simulink model "narmaL2"  (R2017a)
settings: Solver=ode45  StartTime=0.0  StopTime=600  RelTol=1e-3  AbsTol=1e-8  EnableMultiTasking=on
undefined symbols (not defined in the file): Ar, hmax, k12, k2, qmax, qmin
libraries: neural x1
settings Model: Creator=Adolfo  LastModifiedBy=bad
settings DataIOCC: LimitDataPoints=on  SaveFormat=Array  SignalLoggingSaveFormat=ModelDataLogs
settings OptimizationCC: ExpressionDepthLimit=2147483647  InitFltsAndDblsToZero=on  LifeSpan=inf
settings DebuggingCC: SaveWithParameterizedLinksMsg=none  UnderspecifiedInitializationDetection=Classic  MergeDetectMultiDrivingBlocksExec=none  SignalResolutionControl=TryResolveAllWithWarning  SolverPrmCheckMsg=warning  MultiTaskDSMMsg=warning  MultiTaskCondExecSysMsg=none  FcnCallInpInsideContextMsg=warning  StateNameClashWarn=warning  SFUnexpectedBacktrackingDiag=warning  SFNoUnconditionalDefaultTransitionDiag=warning  SFExecutionAtInitializationDiag=none
settings HardwareCC: ProdBitPerPointer=32  ProdBitPerSizeT=32  ProdBitPerPtrDiffT=32  ProdLargestAtomicFloat=None  ProdIntDivRoundTo=Undefined  ProdEndianess=Unspecified  ProdWordSize=32  ProdHWDeviceType=32-bit Generic
settings ModelReferenceCC: PropagateSignalLabelsOutOfModel=off
settings GRTTargetCC: TargetFcnLib=ansi_tfl_tmw.mat  TargetLangStandard=C89/C90 (ANSI)  GeneratePreprocessorConditionals=Disable all  CombineOutputUpdateFcns=off  GRTInterface=on
settings ConfigComp: CovMetricSettings=dw  CovHtmlReporting=on  CovSaveCumulativeToWorkspaceVar=on  CovSaveSingleToWorkspaceVar=on  CovExternalEMLEnable=off

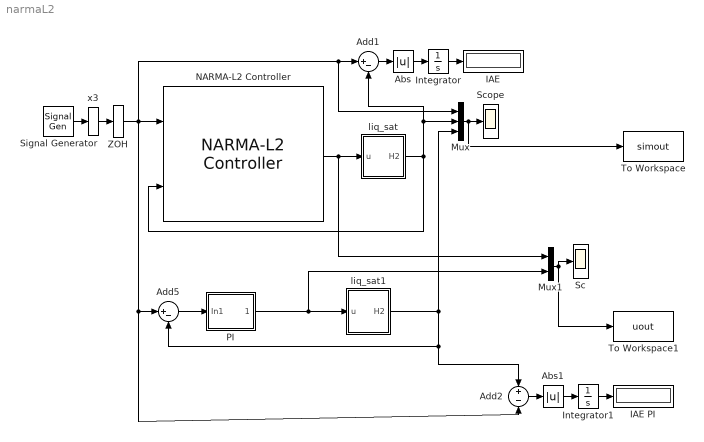
== system narmaL2 ==
  Abs : Abs
  Abs1 : Abs
  Add1 : Sum  Inputs=|+-
  Add2 : Sum  Inputs=+-
  Add5 : Sum  Inputs=|+-
  IAE : Display
  IAE PI : Display
  Integrator : Integrator
  Integrator1 : Integrator
  Mux : Mux  Inputs=3
  Mux1 : Mux  Inputs=2
  NARMA-L2 Controller : neural/Control Systems/NARMA-L2 Controller  Normalize=0  IW1_1=[0.82460127400622895699 0.8896463368737389521 0.68546670272826126791 0.40062646320525224786 -0.25514938442817886033 -1.0240928312478898565 0.01985610351462809009 -0.46086785635635324487 0.94631219312424474932;0.036728497037354770893 0.19820587025539637693 0.5134046067190429774 -0.28308665590364079367 0.16634615705465116697 -0.19327214150223945288 0.44626445203043108023 -0.37497664913527994912 -1.2593297879998377464;0.17045653362356394389 0.023322745585506728799 -0.16838760773330646581 -0.10701132675338295708 0.010654227345909813435 0.1449966612244368569 -0.17756301718275338541 -0.18227958909014374544 -0.38348992703727546871;0.12615415324788967211 -0.18534569723836363808 -1.0200895437469548188 0.76838532857597940939 0.98097883267960284126 -0.21973584499459244967 0.03310600597960997038 0.069654714512501686441 -0.14027211700811134665;0.1320897113109678056 0.31680147111401896209 0.25021595234304006006 -0.016525321314774212705 -0.21919505774665110076 -0.37402348708549482126 -1.0968105491481070501 0.91582443973852623031 0.0044695347566739282094;-0.7988884883001775572 0.77582113437411803769 -0.60287216812896193829 -0.36912054169125485537 0.21145344175312599799 0.041615517227819698309 -0.085528912678096744027 -0.087132152123573891611 0.22015982561206209889;0.38811289402447946006 -0.47324853510461034611 -0.3049238130253699719 0.18104699279980657201 -0.043398814371963738423 1.5082749992737731759 -0.21608774779125763943 -0.2687124972395262823 0.054263947622901022305;1.1246575579809743317 -1.4157437079060470886 0.50688303082942087752 -0.11200608235320431982 -0.019230053512198676258 0.039154841142778194774 -0.020848842953317365395 -0.0039643054993909083994 0.0021401530759821811578;-0.33909893220812831194 0.50899750059057413676 -0.11735584324002928946 -0.019827280110979929317 0.032300329714020560579 -0.024097353999024410248 0.010017402098296960752 0.0026810266030865173396 -0.0014331156384576751797;-1.0805049007907001624 -0.70717796914684893927 0.080234787439031840517 -0.024130003005768181634 0.61532233525059065737 -0.78459118241978287323 -0.35469066371022112127 0.26370174065851531564 0.96317052346297893362;1.9740765052747122343 -1.3610397597231203015 -1.0022880825653401882 -1.0625792463000296451 0.39565868260919517807 1.0051796856926122903 -0.093110283049667660893 0.082619795370768994713 0.016167328722534651808;-0.099469418461439612633 -0.40278027465848725841 -0.47089352901982867161 0.067031861646037194102 0.067547876656573649368 -0.25337998905188230392 0.96800361382420307965 0.45478805765030561048 -0.88698458107894961877;-1.4529527791908256606 0.1568067925322553513 -1.0986307740376015651 0.50153125106809171019 1.8691578273410005551 -0.79110151965966046816 0.73146402793697962164 0.022439777516628570814 0.020810924991256300742;-0.50900373914479313253 0.45814995583261830525 1.1456276180888709249 -1.5430241957026751276 -1.1310824923962929933 1.6740042919720710124 0.0049835931941092440067 -0.21304497923218682076 0.22522168568231107355;-0.37853429671826843705 0.37147006156279560596 -0.039743427633454841974 -0.061152055209479534714 0.042323568373044434532 -0.030245584846645769822 0.0069853908900416143701 0.003085405104233879172 -0.0018039537708811155189]  IW3_2=[-0.0097959372062227899336 0.50164014031742043542 0.63468394272614803153 0.43785446437782760132 -0.85838662096177431593 -1.6429674363166957285 0.18620560020054865991 -0.20320963371365138861 0.1422464600996860562;0.61697123621765026513 -0.88474969392431768167 -0.17864680986586969902 0.57991588808705751834 -0.49305615632303451124 -0.14794008742070452467 -0.03381079823533119505 0.19828324754626353021 -0.13441497495430421161;0.75398603138863662387 -0.48502308801037824493 0.003517610550923244532 0.26274238746623168606 1.5420625628861919232 0.63856894885611914514 -0.96123455216385822464 0.36018548400164290824 0.27701194349752655821;-0.91051269616708951915 -0.33958428131669032846 0.95290714037654755675 0.073612967304474821728 0.20996630936475935147 -0.11065462514984893139 0.077052212643874129494 0.01070943416917579695 -0.012385540173234274586;0.16443588781347087679 0.67006770786870961665 0.6884708055347915634 0.12870790339816937098 -0.41100084195716968249 0.15755452730655974958 -0.73654367631738970612 0.68488352611535630032 0.12549502724547745292;0.96063218759521951107 0.42758867397607214222 -1.2651835130708153354 -0.71554516783911048528 0.33759670629329363578 3.0872236638658465679 -0.25695606251724467661 -0.6782830882585768606 0.30962652904977577828;0.46706721394832628746 0.55353287601559852948 0.69911433634345299115 -0.847525649008489812 -0.25054686095300104931 0.14274435057194184706 -0.18615252503951984497 0.043140727653120047869 0.018608224525331850535;0.8450107012365678516 -1.0798938373582389616 0.4910317222187983166 -0.86347129900768826438 1.0710687752896397296 0.43791333647511820892 0.19374518879967442264 0.075971376265251508442 -0.26660867173805530284;-1.1018119121817588901 -1.4733616883621358795 1.6692288626171432053 0.21358701221124865022 0.043292338661919220477 0.68525051125483049663 0.17902788630519350654 0.23583551788146939199 -0.067173883509847112649;-1.6739081117719991632 1.1177760431219634363 0.47132218615963206165 0.71906947248461727806 -0.42506946994967831355 -2.6242730123560318312 -0.069469553526874824878 0.36308679776155350361 -0.093452349928687061809;-0.77782044035700470541 1.3269413258585924797 -0.43742364026979768665 -0.023010647734847556461 0.017468313680051351239 -0.0088931212673651737627 0.015187382276087291189 0.0036293475455048841011 -0.002197602546328692244;0.11474360757461192495 0.17241811619609576089 -0.19699798228017731394 -0.41145992998582819888 0.37195555743245412028 0.78015868587050629657 0.25978078167190638004 -0.052543511873452151961 -0.25085985498759311163;0.19472679919234092694 0.063155605684590970794 0.13947613217810500563 0.42627460857168703035 0.68910375257047229436 0.43623001225915630785 -0.11874103010955096293 -0.64467095432470289396 0.48229399541859729883;-0.24262201049709156142 -0.95726247674483733174 -0.31738687796607734093 0.56125633081053638573 0.18291069266519230374 0.78624661233304093955 0.16104772558408494976 -0.12893771517534594051 0.085536694064360610512;-0.55990960267259715089 -0.53748643019794273279 -0.63104960549687771909 -0.32569970560154087869 1.0555322514736951156 1.9557692781627589174 0.025912193569968444001 -0.18764326359315686155 0.24956092961725520607]  IW5_3=0.68524973220823459652  LW2_1=[-0.0054733723167232038731 -0.00038308706690342838111 -3.226054861273406793 -0.016004996836879566147 -0.0012809543109151791829 -0.016368029407566965505 -0.0087124206960699276253 3.8506501209388175333 4.4555667968943772905 0.011094954468956964161 -0.0085833479102065679545 -0.0092418423406006207366 -0.0049451264862936479202 -0.0061893334728346308116 -2.6958246976005333373]  LW4_3=[0.028079972834746311922 -0.051315817827737732204 -0.034551189640064525199 0.54739593548655518518 -0.0039848899782993999624 0.062479840311507127415 -0.31148225188883132963 0.090811457968386785633 0.39244861710048445369 -0.055740935256777209006 3.1443772355665582374 0.15600293550726590519 0.045291518824843987612 -0.10872040534465723938 -0.082574408180430783344]  LW5_4=0.85969586982774970352  LW6_5=-0.0047523417828097130888  LW6_2=1.8948110178918895485  B1=[2.609276280555262062;-1.2320213949896976491;-3.9434909003037752484;2.874793119567685018;-1.2328773328075881555;1.8055779013625603557;-0.45002402114329781435;-1.6671970183222060147;-0.83092666539152371108;-0.5200700455604239103;1.0092086295426725417;0.11146887685536957524;0.060081093965868637152;-2.7706489596052730207;0.096621077130841129255]  B2=3.6608075484726660953  B3=[4.5710596781173107317;2.8324585755796536368;-2.4590219130384909363;-3.9609042004329078068;-2.4221799788384923424;2.6143622899144527416;-2.9321292083057981515;-2.4696345991319921254;5.2798580443047660182;-2.3707005348991412319;-2.1247598811442802713;-2.5195907464686913002;2.3967992774617044027;-2.1928615878537627282;1.4244475587535136984]  B4=-5.2688140331114352577  Limit_output=1  min_output=0  max_output=16  Use_Previous_Weights=1  Ts=10  S1=15  Ni=4  Nj=6  sim_file=mod_liq2  trainfun=trainlm  Use_validation=1  Use_Testing=1  max_i=90  min_i=0  max_i_int=100  min_i_int=1  sam_training=2500  epochs=500  minp=0.11705118305365247444  maxp=89.953007277230284444  mint=0  maxt=89.953007277230284444
      settings: SourceProductName=Neural Network Toolbox  SourceProductBaseCode=NN
  PI : Subsystem
  Sc : Scope
  Scope : Scope
  Signal Generator : SignalGenerator  WaveForm=square  Amplitude=-12/300  Frequency=1/600
  To Workspace : ToWorkspace  VariableName=simout  SaveFormat=Timeseries  SampleTime=-1
  To Workspace1 : ToWorkspace  VariableName=uout  SaveFormat=Timeseries  SampleTime=-1
  ZOH : ZeroOrderHold  SampleTime=100
  liq_sat : Subsystem
  liq_sat1 : Subsystem
  x3 : Integrator
  wires:
  Mux/1 -> To Workspace/1, Scope/1
  NARMA-L2 Controller/1 -> Mux1/1, liq_sat/1(u)
  PI/1(Out1) -> Mux1/2, liq_sat1/1(u)
  Add5/1 -> PI/1(In1)
  Mux1/1 -> Sc/1, To Workspace1/1
  liq_sat1/1(H2) -> Add2/1, Add5/2, Mux/3
  liq_sat/1(H2) -> Mux/2, Add1/2, NARMA-L2 Controller/2
  Signal Generator/1 -> x3/1
  x3/1 -> ZOH/1
  ZOH/1 -> Add2/2, Add5/1, Mux/1, Add1/1, NARMA-L2 Controller/1
  Add1/1 -> Abs/1
  Abs/1 -> Integrator/1
  Integrator/1 -> IAE/1
  Add2/1 -> Abs1/1
  Abs1/1 -> Integrator1/1
  Integrator1/1 -> IAE PI/1

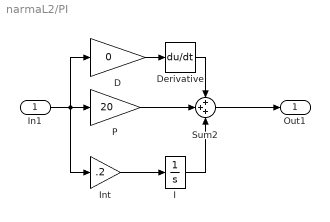
== system narmaL2/PI ==
  In1 : Inport
  D : Gain  Gain=0
  Derivative : Derivative
  I : Integrator
  Int : Gain  Gain=.2
  P : Gain  Gain=20
  Sum2 : Sum  Inputs=+++
  Out1 : Outport
  wires:
  In1/1 -> P/1, Int/1, D/1
  P/1 -> Sum2/2
  I/1 -> Sum2/3
  Sum2/1 -> Out1/1
  Int/1 -> I/1
  D/1 -> Derivative/1
  Derivative/1 -> Sum2/1

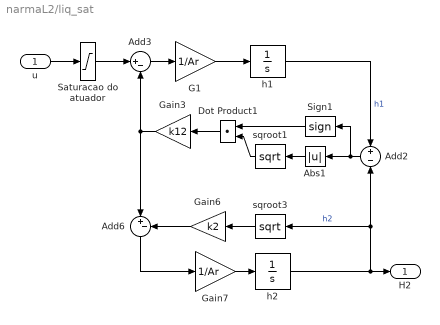
== system narmaL2/liq_sat ==
  u : Inport
  Abs1 : Abs
  Add2 : Sum  Inputs=+-
  Add3 : Sum  Inputs=|+-
  Add6 : Sum  Inputs=|+-
  Dot Product1 : DotProduct  InputSameDT=on  OutDataTypeStr=Inherit: Inherit via internal rule
  G1 : Gain  Gain=1/Ar
  Gain3 : Gain  Gain=k12
  Gain6 : Gain  Gain=k2
  Gain7 : Gain  Gain=1/Ar
  Saturacao do atuador : Saturate  UpperLimit=qmax  LowerLimit=qmin
  Sign1 : Signum
  h1 : Integrator  LimitOutput=on  UpperSaturationLimit=hmax  LowerSaturationLimit=0
  h2 : Integrator  LimitOutput=on  UpperSaturationLimit=hmax  LowerSaturationLimit=0
  sqroot1 : Math  Operator=sqrt  SaturateOnIntegerOverflow=on
  sqroot3 : Math  Operator=sqrt  SaturateOnIntegerOverflow=on
  H2 : Outport
  wires:
  h1/1 -> Add2/1  "h1"
  h2/1 -> Add2/2, sqroot3/1, H2/1  "h2"
  Saturacao do atuador/1 -> Add3/1
  Add6/1 -> Gain7/1
  Gain6/1 -> Add6/2
  Gain7/1 -> h2/1
  sqroot3/1 -> Gain6/1
  G1/1 -> h1/1
  Gain3/1 -> Add6/1, Add3/2
  Add3/1 -> G1/1
  Dot Product1/1 -> Gain3/1
  sqroot1/1 -> Dot Product1/2
  Sign1/1 -> Dot Product1/1
  Abs1/1 -> sqroot1/1
  Add2/1 -> Abs1/1, Sign1/1
  u/1 -> Saturacao do atuador/1

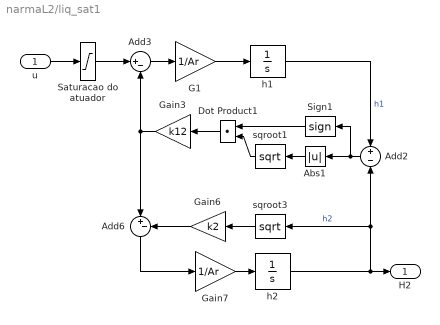
== system narmaL2/liq_sat1 ==
  u : Inport
  Abs1 : Abs
  Add2 : Sum  Inputs=+-
  Add3 : Sum  Inputs=|+-
  Add6 : Sum  Inputs=|+-
  Dot Product1 : DotProduct  InputSameDT=on  OutDataTypeStr=Inherit: Inherit via internal rule
  G1 : Gain  Gain=1/Ar
  Gain3 : Gain  Gain=k12
  Gain6 : Gain  Gain=k2
  Gain7 : Gain  Gain=1/Ar
  Saturacao do atuador : Saturate  UpperLimit=qmax  LowerLimit=qmin
  Sign1 : Signum
  h1 : Integrator  LimitOutput=on  UpperSaturationLimit=hmax  LowerSaturationLimit=0
  h2 : Integrator  LimitOutput=on  UpperSaturationLimit=hmax  LowerSaturationLimit=0
  sqroot1 : Math  Operator=sqrt  SaturateOnIntegerOverflow=on
  sqroot3 : Math  Operator=sqrt  SaturateOnIntegerOverflow=on
  H2 : Outport
  wires:
  h1/1 -> Add2/1  "h1"
  h2/1 -> Add2/2, sqroot3/1, H2/1  "h2"
  Saturacao do atuador/1 -> Add3/1
  Add6/1 -> Gain7/1
  Gain6/1 -> Add6/2
  Gain7/1 -> h2/1
  sqroot3/1 -> Gain6/1
  G1/1 -> h1/1
  Gain3/1 -> Add6/1, Add3/2
  Add3/1 -> G1/1
  Dot Product1/1 -> Gain3/1
  sqroot1/1 -> Dot Product1/2
  Sign1/1 -> Dot Product1/1
  Abs1/1 -> sqroot1/1
  Add2/1 -> Abs1/1, Sign1/1
  u/1 -> Saturacao do atuador/1
